simulink model "voltage_to_kelvin_subsytem"  (R2020b)
settings: Solver=FixedStepAuto  StartTime=0.0  StopTime=10.0  FixedStep=Auto  RelTol=1e-3
libraries: simulink x1
settings Model: Creator=C-TEA  LastModifiedBy=SIRISHA

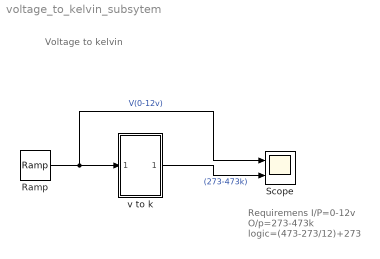
== system voltage_to_kelvin_subsytem ==
  note: Requiremens
      | I/P=0-12v
      | O/p=273-473k
      | logic=(473-273/12)+273
  note: Voltage to kelvin
  Ramp : simulink/Sources/Ramp  slope=1  start=0  InitialOutput=0
  Scope : Scope  NumInputPorts=2
  v to k : Subsystem
  wires:
  Ramp/1 -> Scope/1, v to k/1(In1)  "V(0-12v)"
  v to k/1(Out1) -> Scope/2  "(273-473k)"

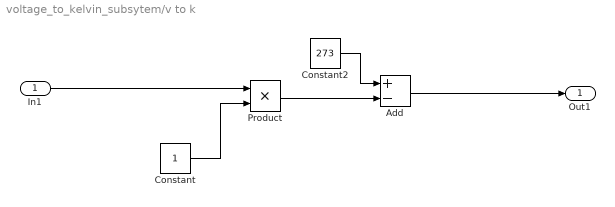
== system voltage_to_kelvin_subsytem/v to k ==
  In1 : Inport
  Add : Sum  Inputs=+-
  Constant : Constant
  Constant2 : Constant  Value=273
  Product : Product
  Out1 : Outport
  wires:
  Constant/1 -> Product/2
  Constant2/1 -> Add/1
  Add/1 -> Out1/1
  Product/1 -> Add/2
  In1/1 -> Product/1
